simulink model "Double_VV"  (R2024a)
settings: Solver=ode1  StartTime=0.0  StopTime=inf  FixedStep=0.01  RelTol=1e-3  EnableMultiTasking=on
settings Model: ExplicitPartitioning=on  Creator=최지웅  LastModifiedBy=최지웅
settings SolverCC: PositivePriorityOrder=on
settings DebuggingCC: AlgebraicLoopMsg=none
settings HardwareCC: ProdBitPerLong=64  ProdHWDeviceType=Intel->x86-64 (Linux 64)
settings RTWCC: Description=Simulink Desktop Real-Time  SystemTargetFile=sldrt.tlc  TemplateMakefile=sldrt.tmf  RTWCompilerOptimization=on  GPUComputeCapability=3.5
settings CodeAppCC: MaxIdLength=95
settings SimulinkDesktopRealTimeCC: TargetLibSuffix=_sldrt.a  TargetPreCompLibLocation=C:\Program Files\MATLAB\R2024a\toolbox\sldrt\lib\win64

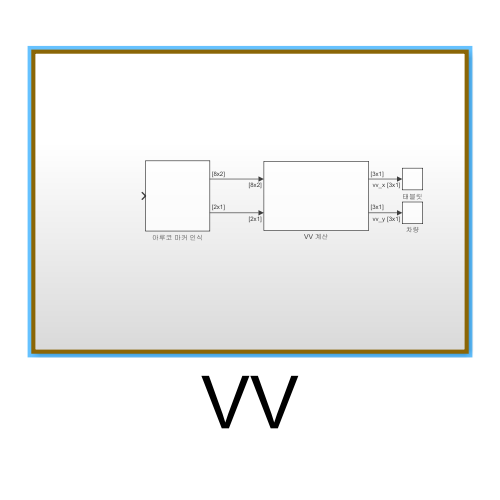
[thumbnail: Simulink's stored preview of the top-level diagram]
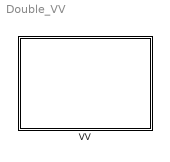
== system Double_VV ==
  VV : Subsystem

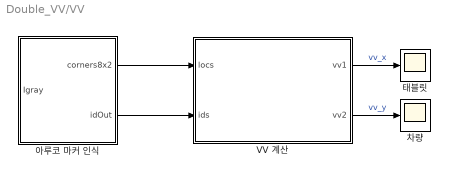
== system Double_VV/VV ==
  VV 계산 : MATLAB Function  TreatAsAtomicUnit=on
  아루코 마커 인식 : MATLAB Function  TreatAsAtomicUnit=on
  차량 : Scope
  태블릿 : Scope
  wires:
  아루코 마커 인식/2(idOut) -> VV 계산/2(ids)
  아루코 마커 인식/1(corners8x2) -> VV 계산/1(locs)
  VV 계산/1(vv1) -> 태블릿/1  "vv_x"
  VV 계산/2(vv2) -> 차량/1  "vv_y"

== matlab function Double_VV/VV/아루코 마커 인식 ==
  data: Igray input; corners8x2 output; idOut output
function [corners8x2, idOut] = fcn(Igray)
% Detect up to two ArUco markers (6×6_250 and 5×5_1000)
%   Igray       : uint8 [H×W] grayscale image
%   corners8x2  : double [8×2] up to 두 개 마커의 네 꼭짓점 (각 마커마다 4×2)
%                 → 첫 4행: 첫 번째 마커, 다음 4행: 두 번째 마커
%   idOut       : uint16 [2×1] 검출된 마커 ID (없으면 0)
%
% R2024a 이상 환경에서 동작

    %#codegen
    coder.extrinsic('readArucoMarker');

    % 출력 초기화
    corners8x2 = zeros(8,2);
    idOut      = uint16([0;0]);

    if isempty(Igray)
        return;
    end

    % 1) 6×6_250 디지털 인식
    [ids6, loc6] = readArucoMarker(Igray, "DICT_6X6_250");
    % 2) 5×5_1000 디지털 인식
    [ids5, loc5] = readArucoMarker(Igray, "DICT_5X5_1000");

    % 합치기
    idsAll = [ids6; ids5];
    locsAll = cat(3, loc6, loc5);  % loc6, loc5 크기: [4×2×N]

    if isempty(idsAll)
        return;
    end

    % 최대 두 개만
    nDetected = min(2, numel(idsAll));
    for idx = 1:nDetected
        idOut(idx) = uint16(idsAll(idx));
        % locsAll(:,:,idx) 는 [4×2]
        corners8x2((idx-1)*4 + (1:4), :) = locsAll(:,:,idx);
    end
end

== matlab function Double_VV/VV/VV 계산 ==
  data: locs input; vv1 output; ids input; vv2 output
function [vv1, vv2] = tiltVV(locs, ids)
% Computes VV vectors for up to two detected ArUco markers
%
% locs : [4×2×N] double – 각 마커의 네 꼭짓점 좌표 (x,y)
% ids  : [N×1] uint16    – 각 마커의 ID
%
% vv1, vv2 : [3×1] double – 첫 번째/두 번째 마커에 대한 VV 벡터 성분
%                         (각각 [vvx; vvy; vvz])
%
% If fewer than two markers are detected, the remaining vv is [0;0;0].

    % 중력가속도
    g = 9.81;
    
    % 초기화
    vv1 = zeros(3,1);
    vv2 = zeros(3,1);
    
    % 검출된 마커가 없으면 바로 리턴
    if isempty(ids)
        return;
    end
    
    % 처리할 마커 수: 최대 2개
    nUse = min(2, numel(ids));
    
    for idx = 1:nUse
        % idx 번째 마커의 네 꼭짓점
        corners = locs(:,:,idx);  % [4×2]
        x1 = corners(1,1);  y1 = corners(1,2);  % top-left
        x2 = corners(2,1);  y2 = corners(2,2);  % top-right
        
        % 화면좌표계 기준 dx, dy
        dx = double(x2 - x1);
        dy = double(y2 - y1);
        
        % raw angle (0~360도)
        raw_rad   = atan2(dy, dx);
        raw_deg   = rad2deg(raw_rad);
        raw_angle = mod(raw_deg + 360, 360);
        
        % tilt (0~180도)
        tmp = mod(90 - raw_angle + 360, 360);
        if tmp > 180
            tilt = 360 - tmp;
        else
            tilt = tmp;
        end
        
        % tilt → 라디안
        theta = deg2rad(tilt);
        
        % VV 벡터 ([vvx; vvy; vvz])
        vv = [ g*cos(theta);
               g*sin(theta);
               0             ];
        
        % 결과 할당
        if idx == 1
            vv1 = vv;
        else
            vv2 = vv;
        end
    end
end
